simulink model "s20260507_5_PIDAdConfig_IMU_quadleg"  (R2025a)
settings: Solver=FixedStepAuto  StartTime=0.0  StopTime=inf  FixedStep=1/100  RelTol=1e-3
undefined symbols (not defined in the file or in its folder): leg1_config, National_Instruments, PCI
libraries: slpidlib x4, sldrtlib x3, simulink x3, cstblocks x2, hostiolib x1, dspstat3 x1
settings Model: Creator=dperera  LastModifiedBy=dperera
settings RTWCC: GPUComputeCapability=3.5

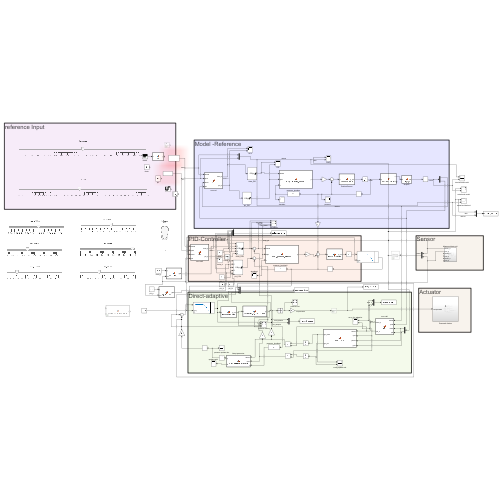
[thumbnail: Simulink's stored preview of the top-level diagram]
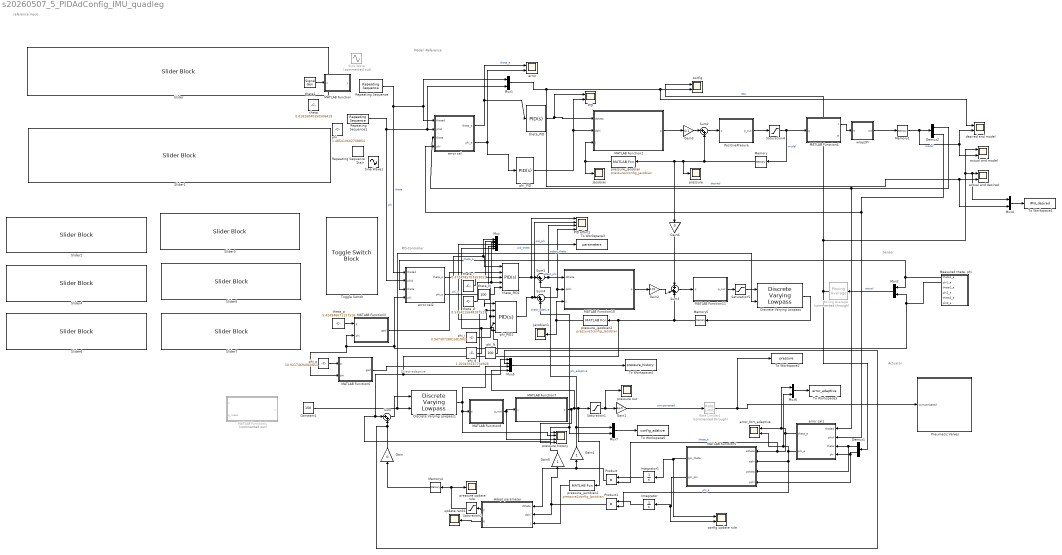
== system s20260507_5_PIDAdConfig_IMU_quadleg ==
  note: reference Input
  note: Actuator
  note: Sensor
  note: Direct-adaptive
  note: PID-Controller
  note: Model -Reference
  Adapt parameter : MATLAB Function  TreatAsAtomicUnit=on
  Constant1 : Constant  Value=150
  Demux1 : Demux  Outputs=2
  Demux2 : Demux  Outputs=2
  Discrete Varying Lowpass : cstblocks/Linear Parameter Varying/Discrete Varying Lowpass  N=1  w0=0  Ts=0.01
  Discrete Varying Lowpass1 : cstblocks/Linear Parameter Varying/Discrete Varying Lowpass  N=1  w0=0  Ts=0.01
  Gain : Gain  Gain=0
  Gain1 : Gain  Gain=1e-5
  Gain2 : Gain  Gain=0.01
  Gain3 : Gain  Gain=0.1
  Gain4 : Gain
  Gain5 : Gain
  Gain6 : Gain  Gain=0
  Integrator : Integrator
  Integrator1 : Integrator
  Jacobian : Scope
      settings: ActiveDisplayYMinimum=-10.825317547305481  ActiveDisplayYMaximum=10.825317547305481  DataLoggingVariableName=ScopeData3
  Jacobian1 : Scope
      settings: ActiveDisplayYMinimum=2.9313515311840069E-6  ActiveDisplayYMaximum=8.8531848611833131E-5  DataLoggingVariableName=ScopeData15
  MATLAB Function : MATLAB Function  TreatAsAtomicUnit=on
  MATLAB Function1 : MATLAB Function  Commented=on  TreatAsAtomicUnit=on
  MATLAB Function10 : MATLAB Function  TreatAsAtomicUnit=on
  MATLAB Function11 : MATLAB Function  TreatAsAtomicUnit=on
  MATLAB Function2 : MATLAB Function  TreatAsAtomicUnit=on
  MATLAB Function3 : MATLAB Function  TreatAsAtomicUnit=on
  MATLAB Function4 : MATLAB Function  TreatAsAtomicUnit=on
  MATLAB Function5 : MATLAB Function  TreatAsAtomicUnit=on
  MATLAB Function6 : MATLAB Function  TreatAsAtomicUnit=on
  MATLAB Function7 : MATLAB Function  TreatAsAtomicUnit=on
  MATLAB Function8 : MATLAB Function  TreatAsAtomicUnit=on
  "Measured theta, phi" : Subsystem
  Memory : Memory  InitialCondition=[1; 1.1; 1]  LinearizeMemory=on  LinearizeAsDelay=on
  Memory1 : Memory  InitialCondition=[0.0001, 0.0001]  LinearizeMemory=on  LinearizeAsDelay=on
  Memory4 : Memory  InitialCondition=[0; 0; 0]
  Memory5 : Memory  InitialCondition=[1; 1.1; 1]  LinearizeMemory=on  LinearizeAsDelay=on
  Moving Average : dspstat3/Moving Average  Commented=through  Method=Sliding window  ForgettingFactorPort=off  SpecifyWindowLength=on  WindowLength=4  OverlapLength=3  AllowArbitraryInputLength=off  ForgettingFactor=0.9  SimulateUsing=Interpreted execution
  Mux : Mux  Inputs=6
  Mux{1..2,4,6..7} (5 alike) : Mux  Inputs=2
  Mux5 : Mux
  PID : Scope  NumInputPorts=2
      settings: ActiveDisplayYMinimum=-3.9804584732791981  ActiveDisplayYMaximum=3.8453740981888478  DataLoggingVariableName=ScopeData4
  PID efforts : Scope  NumInputPorts=4
      settings: ActiveDisplayYMinimum=-41.407944293192642  ActiveDisplayYMaximum=165.36846848361682  DataLoggingVariableName=ScopeData5
  Pneumatic Valves : Subsystem
  PositivePresure : MATLAB Function  TreatAsAtomicUnit=on
  Product : Product
  Product1 : Product
  Rate Limiter1 : RateLimiter  Commented=through  SampleTimeMode=inherited
  Repeating Sequence : simulink/Sources/Repeating Sequence  rep_seq_t=t  rep_seq_y=leg1_config(1,:)
  Repeating Sequence Stair : simulink/Sources/Repeating Sequence Stair  OutValues=[1.1 1.6].'  tsamp=1  OutMin=[]  OutMax=[]  OutDataTypeStr=double  OutputDataTypeScalingMode=double  OutDataType=fixdt(0,8)  ConRadixGroup=Best Precision: Vector-wise  OutScaling=2^-12
  Repeating Sequence1 : simulink/Sources/Repeating Sequence  rep_seq_t=t  rep_seq_y=leg1_config(2,:)
  Saturation{1..2,4..5} (4 alike) : Saturate  UpperLimit=300000  LowerLimit=0
  Sine Wave : Sin  Commented=on  Amplitude=0.2  Frequency=1/2  SampleTime=0
  Sine Wave1 : Sin  Amplitude=1.5/4  Bias=1  Frequency=0.5  SampleTime=0
  Slider : SliderBlock  ScaleMin=-3.14  ScaleMax=3.14
  Slider1 : SliderBlock  ScaleMax=3.14
  Slider2 : SliderBlock  ScaleMax=10
  Slider3 : SliderBlock  ScaleMax=20
  Slider4 : SliderBlock  ScaleMax=1
  Slider5 : SliderBlock  ScaleMax=1
  Slider6 : SliderBlock  ScaleMax=3
  Slider7 : SliderBlock  ScaleMax=3
  Sum{,1..2,4} (4 alike) : Sum  Inputs=|++
  Sum3 : Sum  Inputs=+|++
  To Workspace1 : ToWorkspace  VariableName=IMU_desired  SaveFormat=Timeseries  SampleTime=-1
  To Workspace2 : ToWorkspace  VariableName=pressure  SaveFormat=Timeseries  SampleTime=-1
  To Workspace3 : ToWorkspace  VariableName=parameters  SaveFormat=Timeseries  SampleTime=-1
  To Workspace4 : ToWorkspace  VariableName=pressure_history  SaveFormat=Timeseries  SampleTime=-1
  To Workspace5 : ToWorkspace  VariableName=error_adaptive  SaveFormat=Timeseries  SampleTime=-1
  To Workspace6 : ToWorkspace  VariableName=config_adative  SaveFormat=Timeseries  SampleTime=-1
  Toggle Switch : ToggleSwitchBlock
  actual and desired : Scope  NumInputPorts=2
      settings: ActiveDisplayYMinimum=-3.9267574076576723  ActiveDisplayYMaximum=3.9248901330211212  DataLoggingVariableName=ScopeData8
  actual and model : Scope  NumInputPorts=2
      settings: ActiveDisplayYMinimum=-2.3315152827249515  ActiveDisplayYMaximum=2.6797978799735036  DataLoggingVariableName=ScopeData16
  config : Scope  NumInputPorts=2
      settings: ActiveDisplayYMinimum=-3.926205418823844  ActiveDisplayYMaximum=3.9199222335166648
  config update rule : Scope  NumInputPorts=2
      settings: ActiveDisplayYMinimum=-0.92286339962463748  ActiveDisplayYMaximum=0.53131241193978052  DataLoggingVariableName=ScopeData13
  desired and model : Scope  NumInputPorts=2
      settings: ActiveDisplayYMinimum=-3.9267537424057748  ActiveDisplayYMaximum=3.9248571457540451  DataLoggingVariableName=ScopeData14
  error : Scope  NumInputPorts=2
      settings: ActiveDisplayYMinimum=-1.7062614665873941  ActiveDisplayYMaximum=3.7647403361072445
  error cal : MATLAB Function  TreatAsAtomicUnit=on
  error cal1 : MATLAB Function  TreatAsAtomicUnit=on
  error cal2 : MATLAB Function  TreatAsAtomicUnit=on
  error_fort_adaptive : Scope  NumInputPorts=2
      settings: ActiveDisplayYMinimum=-2.3074635708077071  ActiveDisplayYMaximum=1.3880246681318078  DataLoggingVariableName=ScopeData11
  phi : Constant  Value=1.485410602708854
  phi_N : Constant  Value=100
  phi_PID : slpidlib/PID Controller  Controller=PID  Form=Parallel  TimeDomain=Continuous-time  UseExternalTs=off  SampleTime=-1  IntegratorMethod=Forward Euler  FilterMethod=Forward Euler  ControllerParametersSource=internal  P=10  I=0.5  UseKiTs=off  D=0.01  UseExternalDerivativeSource=off  N=100  UseFilter=on  TunerSelectOption=Transfer Function Based (PID Tuner App)  InitialConditionSource=internal  InitialConditionForIntegrator=0  InitialConditionForFilter=0  DifferentiatorICPrevScaledInput=0  ExternalReset=none  TrackingMode=off  Kt=1  LimitOutput=on  SatLimitsSource=internal  UpperSaturationLimit=inf  LowerSaturationLimit=-inf  LinearizeAsGain=off  AntiWindupMode=back-calculation  Kb=1  LimitIntegrator=off  UpperIntegratorSaturationLimit=10  LowerIntegratorSaturationLimit=-10  POutMin=[]  POutMax=[]  IOutMin=[]  IOutMax=[]  DOutMin=[]  DOutMax=[]  NOutMin=[]  NOutMax=[]  SumOutMin=[]  SumOutMax=[]  SaturationOutMin=[]  SaturationOutMax=[]  PParamMin=[]  PParamMax=[]  IParamMin=[]  IParamMax=[]  DParamMin=[]  DParamMax=[]  NParamMin=[]  NParamMax=[]  KbParamMin=[]  KbParamMax=[]  KtParamMin=[]  KtParamMax=[]  KbOutMin=[]  KbOutMax=[]  KtOutMin=[]  KtOutMax=[]  IntegratorOutMin=[]  IntegratorOutMax=[]  FilterOutMin=[]  FilterOutMax=[]  SumI1OutMin=[]  SumI1OutMax=[]  SumI2OutMin=[]  SumI2OutMax=[]  SumI3OutMin=[]  SumI3OutMax=[]  SumI4OutMin=[]  SumI4OutMax=[]  SumDOutMin=[]  SumDOutMax=[]  DifferentiatorOutMin=[]  DifferentiatorOutMax=[]  FilterDiffOutCoefMin=[]  FilterDiffOutCoefMax=[]  ReciprocalOutMin=[]  ReciprocalOutMax=[]  SumDenOutMin=[]  SumDenOutMax=[]  SumNumOutMin=[]  SumNumOutMax=[]  DivideOutMin=[]  DivideOutMax=[]  UdiffTsProdOutMin=[]  UdiffTsProdOutMax=[]  NTsProdOutMin=[]  NTsProdOutMax=[]  UintegralTsProdOutMin=[]  UintegralTsProdOutMax=[]  UngainTsProdOutMin=[]  UngainTsProdOutMax=[]  ClampingZeroOutDataTypeStr=Inherit: Inherit via back propagation  ClampingZeroOutMin=[]  ClampingZeroOutMax=[]  FilterDenConstantOutDataTypeStr=Inherit: Inherit via back propagation  FilterDenConstantOutMin=[]  FilterDenConstantOutMax=[]  PCopyOutDataTypeStr=Inherit: Inherit via back propagation  PCopyOutMin=[]  PCopyOutMax=[]  NCopyOutDataTypeStr=Inherit: Inherit via back propagation  NCopyOutMin=[]  NCopyOutMax=[]  IntegratorContinuousStateAttributes=''  IntegratorStateMustResolveToSignalObject=off  IntegratorRTWStateStorageClass=Auto  FilterContinuousStateAttributes=''  FilterStateMustResolveToSignalObject=off  FilterRTWStateStorageClass=Auto  ParallelPVariant=InternalParameters  IdealPVariant=Disabled  IVariant=InternalParameters  DVariant=InternalParameters  IntegratorVariant=Continuous  SatVariant=Enabled  AWVariant=BackCalculation  PCopyVariant=Disabled  TRVariant=Disabled  FdbkBlocksVariant=Forward  IdealPFdbkVariant=Disabled  SatFdbkVariant=Disabled  DerivativeFilterVariant=ContFilter  NVariant=InternalParameters  NCopyVariant=Disabled  FilterICVariant=InternalICsFilter  IntegratorICVariant=InternalICs  ExternalResetVariant=Disabled  TRSumVariant=Passthrough  SumFdbkVariant=Disabled  SumVariant=Sum_PID  TsampFilterVariant=InternalTs  TsampNgainVariant=Passthrough  TsampIntegralVariant=Disabled_SignalSpec  ExternalSaturationOutDataTypeStr=Inherit: Same as second input  DerivativeSourceVariant=ErrorSignal  PreIntVariant=InternalPreInt
  phi_PID1 : slpidlib/PID Controller  Controller=PID  Form=Parallel  TimeDomain=Continuous-time  UseExternalTs=off  SampleTime=-1  IntegratorMethod=Forward Euler  FilterMethod=Forward Euler  ControllerParametersSource=external  P=3.5  I=0.01  UseKiTs=off  D=0.02  UseExternalDerivativeSource=off  N=100  UseFilter=on  TunerSelectOption=Transfer Function Based (PID Tuner App)  InitialConditionSource=internal  InitialConditionForIntegrator=0  InitialConditionForFilter=0  DifferentiatorICPrevScaledInput=0  ExternalReset=none  TrackingMode=off  Kt=1  LimitOutput=on  SatLimitsSource=internal  UpperSaturationLimit=inf  LowerSaturationLimit=-inf  LinearizeAsGain=off  AntiWindupMode=back-calculation  Kb=2  LimitIntegrator=off  UpperIntegratorSaturationLimit=10  LowerIntegratorSaturationLimit=-10  POutMin=[]  POutMax=[]  IOutMin=[]  IOutMax=[]  DOutMin=[]  DOutMax=[]  NOutMin=[]  NOutMax=[]  SumOutMin=[]  SumOutMax=[]  SaturationOutMin=[]  SaturationOutMax=[]  PParamMin=[]  PParamMax=[]  IParamMin=[]  IParamMax=[]  DParamMin=[]  DParamMax=[]  NParamMin=[]  NParamMax=[]  KbParamMin=[]  KbParamMax=[]  KtParamMin=[]  KtParamMax=[]  KbOutMin=[]  KbOutMax=[]  KtOutMin=[]  KtOutMax=[]  IntegratorOutMin=[]  IntegratorOutMax=[]  FilterOutMin=[]  FilterOutMax=[]  SumI1OutMin=[]  SumI1OutMax=[]  SumI2OutMin=[]  SumI2OutMax=[]  SumI3OutMin=[]  SumI3OutMax=[]  SumI4OutMin=[]  SumI4OutMax=[]  SumDOutMin=[]  SumDOutMax=[]  DifferentiatorOutMin=[]  DifferentiatorOutMax=[]  FilterDiffOutCoefMin=[]  FilterDiffOutCoefMax=[]  ReciprocalOutMin=[]  ReciprocalOutMax=[]  SumDenOutMin=[]  SumDenOutMax=[]  SumNumOutMin=[]  SumNumOutMax=[]  DivideOutMin=[]  DivideOutMax=[]  UdiffTsProdOutMin=[]  UdiffTsProdOutMax=[]  NTsProdOutMin=[]  NTsProdOutMax=[]  UintegralTsProdOutMin=[]  UintegralTsProdOutMax=[]  UngainTsProdOutMin=[]  UngainTsProdOutMax=[]  ClampingZeroOutDataTypeStr=Inherit: Inherit via back propagation  ClampingZeroOutMin=[]  ClampingZeroOutMax=[]  FilterDenConstantOutDataTypeStr=Inherit: Inherit via back propagation  FilterDenConstantOutMin=[]  FilterDenConstantOutMax=[]  PCopyOutDataTypeStr=Inherit: Inherit via back propagation  PCopyOutMin=[]  PCopyOutMax=[]  NCopyOutDataTypeStr=Inherit: Inherit via back propagation  NCopyOutMin=[]  NCopyOutMax=[]  IntegratorContinuousStateAttributes=''  IntegratorStateMustResolveToSignalObject=off  IntegratorRTWStateStorageClass=Auto  FilterContinuousStateAttributes=''  FilterStateMustResolveToSignalObject=off  FilterRTWStateStorageClass=Auto  ParallelPVariant=ExternalParameters  IdealPVariant=Disabled  IVariant=ExternalParameters  DVariant=ExternalParameters  IntegratorVariant=Continuous  SatVariant=Enabled  AWVariant=BackCalculation  PCopyVariant=Disabled  TRVariant=Disabled  FdbkBlocksVariant=Forward  IdealPFdbkVariant=Disabled  SatFdbkVariant=Disabled  DerivativeFilterVariant=ContFilter  NVariant=ExternalParameters  NCopyVariant=Disabled  FilterICVariant=InternalICsFilter  IntegratorICVariant=InternalICs  ExternalResetVariant=Disabled  TRSumVariant=Passthrough  SumFdbkVariant=Disabled  SumVariant=Sum_PID  TsampFilterVariant=InternalTs  TsampNgainVariant=Passthrough  TsampIntegralVariant=Disabled_SignalSpec  ExternalSaturationOutDataTypeStr=Inherit: Same as second input  DerivativeSourceVariant=ErrorSignal  PreIntVariant=InternalPreInt
  phi_d : Constant  Value=1.020433147734928
  phi_i : Constant  Value=0.9473072881581902
  phi_p : Constant  Value=10.92174694060851
  pressure : Scope
      settings: ActiveDisplayYMinimum=-37499.999999999993  ActiveDisplayYMaximum=337500  DataLoggingVariableName=ScopeData2
  pressure history : Scope  NumInputPorts=4
      settings: ActiveDisplayYMinimum=-38849.124995166283  ActiveDisplayYMaximum=349642.12495649664  DataLoggingVariableName=ScopeData17
  pressure out : Scope
      settings: ActiveDisplayYMinimum=-37499.999999999993  ActiveDisplayYMaximum=337500  DataLoggingVariableName=ScopeData12
  pressure update rule : Scope
      settings: ActiveDisplayYMinimum=-11428.615964886589  ActiveDisplayYMaximum=102857.54368397931  DataLoggingVariableName=ScopeData9
  pressure_jacobian : MATLABFcn  MATLABFcn=pressure2config_Jacobian  OutputDimensions=[2 3]  OutputSignalType=real  Output1D=off
  pressure_jacobian1 : MATLABFcn  MATLABFcn=pressure2config_Jacobian  OutputDimensions=[2 3]  OutputSignalType=real  Output1D=off
  pressure_jacobian2 : MATLABFcn  MATLABFcn=pressure2config_Jacobian  OutputDimensions=[2 3]  OutputSignalType=real  Output1D=off
  theta : Constant  Value=0.01826040350506419
  theta1 : SignalGenerator  WaveForm=sawtooth  Amplitude=pi  Frequency=0.05*2*pi  Units=rad/sec  VectorParams1D=off
  theta_N : Constant  Value=100
  theta_PID : slpidlib/PID Controller  Controller=PID  Form=Parallel  TimeDomain=Continuous-time  UseExternalTs=off  SampleTime=-1  IntegratorMethod=Forward Euler  FilterMethod=Forward Euler  ControllerParametersSource=internal  P=5  I=0.1  UseKiTs=off  D=0  UseExternalDerivativeSource=off  N=100  UseFilter=on  TunerSelectOption=Transfer Function Based (PID Tuner App)  InitialConditionSource=internal  InitialConditionForIntegrator=0  InitialConditionForFilter=0  DifferentiatorICPrevScaledInput=0  ExternalReset=none  TrackingMode=off  Kt=1  LimitOutput=on  SatLimitsSource=internal  UpperSaturationLimit=inf  LowerSaturationLimit=-inf  LinearizeAsGain=off  AntiWindupMode=back-calculation  Kb=1  LimitIntegrator=off  UpperIntegratorSaturationLimit=10  LowerIntegratorSaturationLimit=-10  POutMin=[]  POutMax=[]  IOutMin=[]  IOutMax=[]  DOutMin=[]  DOutMax=[]  NOutMin=[]  NOutMax=[]  SumOutMin=[]  SumOutMax=[]  SaturationOutMin=[]  SaturationOutMax=[]  PParamMin=[]  PParamMax=[]  IParamMin=[]  IParamMax=[]  DParamMin=[]  DParamMax=[]  NParamMin=[]  NParamMax=[]  KbParamMin=[]  KbParamMax=[]  KtParamMin=[]  KtParamMax=[]  KbOutMin=[]  KbOutMax=[]  KtOutMin=[]  KtOutMax=[]  IntegratorOutMin=[]  IntegratorOutMax=[]  FilterOutMin=[]  FilterOutMax=[]  SumI1OutMin=[]  SumI1OutMax=[]  SumI2OutMin=[]  SumI2OutMax=[]  SumI3OutMin=[]  SumI3OutMax=[]  SumI4OutMin=[]  SumI4OutMax=[]  SumDOutMin=[]  SumDOutMax=[]  DifferentiatorOutMin=[]  DifferentiatorOutMax=[]  FilterDiffOutCoefMin=[]  FilterDiffOutCoefMax=[]  ReciprocalOutMin=[]  ReciprocalOutMax=[]  SumDenOutMin=[]  SumDenOutMax=[]  SumNumOutMin=[]  SumNumOutMax=[]  DivideOutMin=[]  DivideOutMax=[]  UdiffTsProdOutMin=[]  UdiffTsProdOutMax=[]  NTsProdOutMin=[]  NTsProdOutMax=[]  UintegralTsProdOutMin=[]  UintegralTsProdOutMax=[]  UngainTsProdOutMin=[]  UngainTsProdOutMax=[]  ClampingZeroOutDataTypeStr=Inherit: Inherit via back propagation  ClampingZeroOutMin=[]  ClampingZeroOutMax=[]  FilterDenConstantOutDataTypeStr=Inherit: Inherit via back propagation  FilterDenConstantOutMin=[]  FilterDenConstantOutMax=[]  PCopyOutDataTypeStr=Inherit: Inherit via back propagation  PCopyOutMin=[]  PCopyOutMax=[]  NCopyOutDataTypeStr=Inherit: Inherit via back propagation  NCopyOutMin=[]  NCopyOutMax=[]  IntegratorContinuousStateAttributes=''  IntegratorStateMustResolveToSignalObject=off  IntegratorRTWStateStorageClass=Auto  FilterContinuousStateAttributes=''  FilterStateMustResolveToSignalObject=off  FilterRTWStateStorageClass=Auto  ParallelPVariant=InternalParameters  IdealPVariant=Disabled  IVariant=InternalParameters  DVariant=InternalParameters  IntegratorVariant=Continuous  SatVariant=Enabled  AWVariant=BackCalculation  PCopyVariant=Disabled  TRVariant=Disabled  FdbkBlocksVariant=Forward  IdealPFdbkVariant=Disabled  SatFdbkVariant=Disabled  DerivativeFilterVariant=ContFilter  NVariant=InternalParameters  NCopyVariant=Disabled  FilterICVariant=InternalICsFilter  IntegratorICVariant=InternalICs  ExternalResetVariant=Disabled  TRSumVariant=Passthrough  SumFdbkVariant=Disabled  SumVariant=Sum_PID  TsampFilterVariant=InternalTs  TsampNgainVariant=Passthrough  TsampIntegralVariant=Disabled_SignalSpec  ExternalSaturationOutDataTypeStr=Inherit: Same as second input  DerivativeSourceVariant=ErrorSignal  PreIntVariant=InternalPreInt
  theta_PID1 : slpidlib/PID Controller  Controller=PID  Form=Parallel  TimeDomain=Continuous-time  UseExternalTs=off  SampleTime=-1  IntegratorMethod=Forward Euler  FilterMethod=Forward Euler  ControllerParametersSource=external  P=3  I=0.1  UseKiTs=off  D=0.001  UseExternalDerivativeSource=off  N=100  UseFilter=on  TunerSelectOption=Transfer Function Based (PID Tuner App)  InitialConditionSource=internal  InitialConditionForIntegrator=0  InitialConditionForFilter=0  DifferentiatorICPrevScaledInput=0  ExternalReset=none  TrackingMode=off  Kt=1  LimitOutput=on  SatLimitsSource=internal  UpperSaturationLimit=inf  LowerSaturationLimit=-inf  LinearizeAsGain=off  AntiWindupMode=back-calculation  Kb=2  LimitIntegrator=off  UpperIntegratorSaturationLimit=10  LowerIntegratorSaturationLimit=-10  POutMin=[]  POutMax=[]  IOutMin=[]  IOutMax=[]  DOutMin=[]  DOutMax=[]  NOutMin=[]  NOutMax=[]  SumOutMin=[]  SumOutMax=[]  SaturationOutMin=[]  SaturationOutMax=[]  PParamMin=[]  PParamMax=[]  IParamMin=[]  IParamMax=[]  DParamMin=[]  DParamMax=[]  NParamMin=[]  NParamMax=[]  KbParamMin=[]  KbParamMax=[]  KtParamMin=[]  KtParamMax=[]  KbOutMin=[]  KbOutMax=[]  KtOutMin=[]  KtOutMax=[]  IntegratorOutMin=[]  IntegratorOutMax=[]  FilterOutMin=[]  FilterOutMax=[]  SumI1OutMin=[]  SumI1OutMax=[]  SumI2OutMin=[]  SumI2OutMax=[]  SumI3OutMin=[]  SumI3OutMax=[]  SumI4OutMin=[]  SumI4OutMax=[]  SumDOutMin=[]  SumDOutMax=[]  DifferentiatorOutMin=[]  DifferentiatorOutMax=[]  FilterDiffOutCoefMin=[]  FilterDiffOutCoefMax=[]  ReciprocalOutMin=[]  ReciprocalOutMax=[]  SumDenOutMin=[]  SumDenOutMax=[]  SumNumOutMin=[]  SumNumOutMax=[]  DivideOutMin=[]  DivideOutMax=[]  UdiffTsProdOutMin=[]  UdiffTsProdOutMax=[]  NTsProdOutMin=[]  NTsProdOutMax=[]  UintegralTsProdOutMin=[]  UintegralTsProdOutMax=[]  UngainTsProdOutMin=[]  UngainTsProdOutMax=[]  ClampingZeroOutDataTypeStr=Inherit: Inherit via back propagation  ClampingZeroOutMin=[]  ClampingZeroOutMax=[]  FilterDenConstantOutDataTypeStr=Inherit: Inherit via back propagation  FilterDenConstantOutMin=[]  FilterDenConstantOutMax=[]  PCopyOutDataTypeStr=Inherit: Inherit via back propagation  PCopyOutMin=[]  PCopyOutMax=[]  NCopyOutDataTypeStr=Inherit: Inherit via back propagation  NCopyOutMin=[]  NCopyOutMax=[]  IntegratorContinuousStateAttributes=''  IntegratorStateMustResolveToSignalObject=off  IntegratorRTWStateStorageClass=Auto  FilterContinuousStateAttributes=''  FilterStateMustResolveToSignalObject=off  FilterRTWStateStorageClass=Auto  ParallelPVariant=ExternalParameters  IdealPVariant=Disabled  IVariant=ExternalParameters  DVariant=ExternalParameters  IntegratorVariant=Continuous  SatVariant=Enabled  AWVariant=BackCalculation  PCopyVariant=Disabled  TRVariant=Disabled  FdbkBlocksVariant=Forward  IdealPFdbkVariant=Disabled  SatFdbkVariant=Disabled  DerivativeFilterVariant=ContFilter  NVariant=ExternalParameters  NCopyVariant=Disabled  FilterICVariant=InternalICsFilter  IntegratorICVariant=InternalICs  ExternalResetVariant=Disabled  TRSumVariant=Passthrough  SumFdbkVariant=Disabled  SumVariant=Sum_PID  TsampFilterVariant=InternalTs  TsampNgainVariant=Passthrough  TsampIntegralVariant=Disabled_SignalSpec  ExternalSaturationOutDataTypeStr=Inherit: Same as second input  DerivativeSourceVariant=ErrorSignal  PreIntVariant=InternalPreInt
  theta_d : Constant  Value=0.5354215648287513
  theta_i : Constant  Value=0.3724785703353051
  theta_p : Constant  Value=5.424946671157516
  update rank1 : Scope
      settings: ActiveDisplayYMinimum=-0.12499999999999997  ActiveDisplayYMaximum=1.125  DataLoggingVariableName=ScopeData10
  wrap2Pi : MATLAB Function  TreatAsAtomicUnit=on
  wires:
  error cal/2(phi_e) -> error/2, phi_PID/1
  pressure_jacobian/1 -> Jacobian/1, MATLAB Function2/3(J)
  theta_PID/1 -> PID/1, MATLAB Function2/1(dtheta)
  phi_PID/1 -> PID/2, MATLAB Function2/2(dphi)
  Memory/1 -> pressure/1, Gain6/1, pressure_jacobian/1, Sum2/2
  Mux1/1 -> desired and model/1, config/2, Mux4/2, actual and desired/2  "desired"
  Gain3/1 -> Sum2/1
  Sum2/1 -> PositivePresure/1(p)
  Saturation4/1 -> MATLAB Function4/1(p), Memory/1  "model"
  MATLAB Function2/1(p) -> Gain3/1
  error cal/1(theta_e) -> error/1, theta_PID/1  "theta_e"
  Mux2/1 -> Moving Average/1  "actual"
  theta1/1 -> MATLAB Function/1(u)
  PositivePresure/1(p_out) -> Saturation4/1
  Integrator1/1 -> Product/1
  Integrator/1 -> Product1/1
  Adapt parameter/1(p) -> Saturation2/1
  Saturation2/1 -> Memory4/1, pressure update rule/1
  error cal1/2(phi_e) -> error_fort_adaptive/2, Mux6/2, Product1/2, MATLAB Function5/2(ephi)  "phi_e"
  pressure_jacobian1/1 -> Adapt parameter/3(J)
  MATLAB Function5/2(gm_phi) -> config update rule/2, Integrator/1
  Product/1 -> Adapt parameter/1(dtheta), Gain4/1
  Demux2/2 -> error cal1/2(phid), error cal/4(phi)
  error cal1/1(theta_e) -> Mux6/1, error_fort_adaptive/1, Product/2, MATLAB Function5/1(etheta)  "theta_e"
  Demux2/1 -> error cal1/1(thetad), error cal/3(theta)
  Product1/1 -> Gain5/1, Adapt parameter/2(dphi)
  Demux1/2 -> MATLAB Function5/4(pphi), error cal1/4(phi)
  Sum/1 -> Discrete Varying Lowpass1/1
  Demux1/1 -> MATLAB Function5/3(ptheta), error cal1/3(theta)
  Gain/1 -> Mux5/2, Sum/2
  Adapt parameter/2(R) -> update rank1/1
  MATLAB Function5/1(gm_theta) -> Integrator1/1, config update rule/1
  wrap2Pi/1(wa) -> Memory1/1
  MATLAB Function4/1(c) -> wrap2Pi/1(a)
  Saturation1/1 -> pressure out/1, Gain1/1
  Gain1/1 -> Rate Limiter1/1  "compensated"
  Memory1/1 -> actual and model/2, desired and model/2, Demux2/1  "model"
  Memory4/1 -> Gain/1
  MATLAB Function11/1(p_out) -> Saturation5/1
  "Measured theta, phi"/1(theta1_a) -> Mux2/1, error cal2/3(theta)
  MATLAB Function10/1(p) -> Gain2/1
  phi_PID1/1 -> PID efforts/2, Sum4/1  "pid_phi"
  error cal2/2(phi_e) -> phi_PID1/1  "phi_e"
  "Measured theta, phi"/2(phi1_a) -> Mux2/2, MATLAB Function6/2(phi), MATLAB Function3/2(phi), error cal2/4(phi)
  Memory5/1 -> Sum3/3, pressure_jacobian2/1, pressure history/1, Sum/1, Mux5/1
  Sum3/1 -> MATLAB Function11/1(p)
  Repeating Sequence/1 -> error cal2/1(thetad), error cal/1(thetad), Mux1/1  "theta"
  pressure_jacobian2/1 -> Jacobian1/1, MATLAB Function10/3(J)
  Saturation5/1 -> Discrete Varying Lowpass/1
  Repeating Sequence1/1 -> error cal2/2(phid), Mux1/2, error cal/2(phid)  "phi"
  error cal2/1(theta_e) -> Mux/1, theta_PID1/1  "theta_e"
  MATLAB Function7/1(p) -> Mux5/4, pressure_jacobian1/1, Saturation1/1, pressure history/4
  MATLAB Function8/1(p_out) -> MATLAB Function7/1(x), pressure history/3
  Moving Average/1 -> actual and model/1, Mux4/1, actual and desired/1, config/1, Demux1/1  "IMU"
  Mux4/1 -> To Workspace1/1
  MATLAB Function6/1(gad) -> Mux/4, phi_PID1/2
  phi_i/1 -> Mux/5, phi_PID1/3
  phi_d/1 -> phi_PID1/4, Mux/6
  phi_N/1 -> phi_PID1/5
  MATLAB Function3/1(gad) -> theta_PID1/2
  theta_i/1 -> Mux/2, theta_PID1/3
  theta_d/1 -> Mux/3, theta_PID1/4
  theta_N/1 -> theta_PID1/5
  theta_p/1 -> MATLAB Function3/1(g)
  phi_p/1 -> MATLAB Function6/1(g)
  Discrete Varying Lowpass/1 -> Memory5/1
  Rate Limiter1/1 -> To Workspace2/1, Pneumatic Valves/1(compensated)
  Mux/1 -> To Workspace3/1
  Mux5/1 -> To Workspace4/1
  theta_PID1/1 -> PID efforts/1, Sum1/1  "pid_theta"
  Sum1/1 -> PID efforts/3, MATLAB Function10/1(dtheta)  "adapt_theta"
  Sum4/1 -> PID efforts/4, MATLAB Function10/2(dphi)  "adapt_phi"
  Gain4/1 -> Mux7/1, Sum1/2  "theta_adative"
  Gain5/1 -> Mux7/2, Sum4/2  "phi_adaptive"
  Constant1/1 -> Discrete Varying Lowpass/2, Discrete Varying Lowpass1/2
  Discrete Varying Lowpass1/1 -> Mux5/3, pressure history/2, MATLAB Function8/1(p)
  Gain2/1 -> Sum3/2
  Gain6/1 -> Sum3/1
  Mux6/1 -> To Workspace5/1
  Mux7/1 -> To Workspace6/1

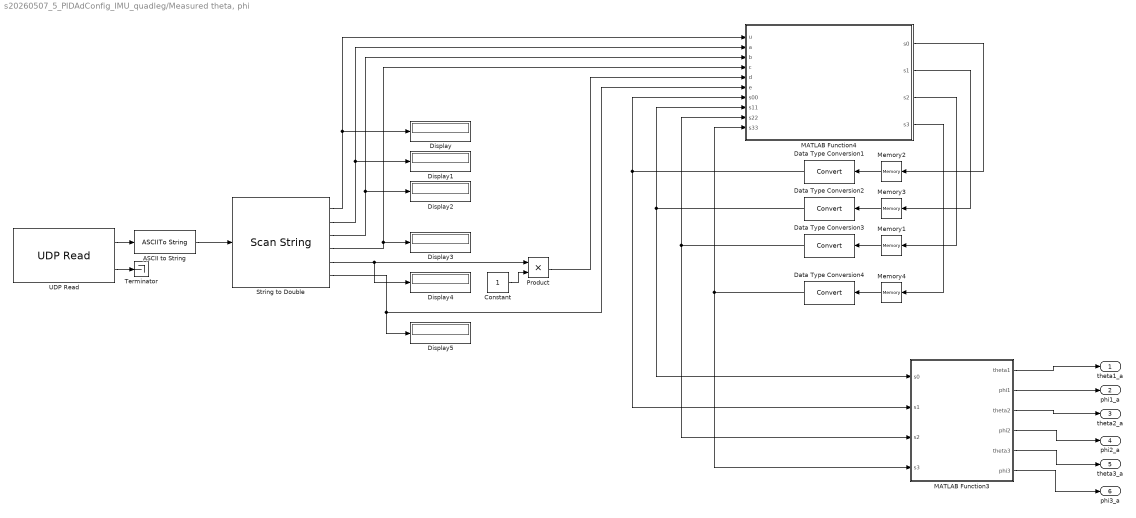
== system s20260507_5_PIDAdConfig_IMU_quadleg/Measured theta, phi ==
  ASCII to String : ASCIIToString
  Constant : Constant
  Data Type Conversion{1..4} (4 alike) : DataTypeConversion  SaturateOnIntegerOverflow=off  RndMeth=Floor
  Display{,1..5} (6 alike) : Display
  MATLAB Function3 : MATLAB Function  TreatAsAtomicUnit=on
  MATLAB Function4 : MATLAB Function  TreatAsAtomicUnit=on
  Memory1 : Memory  InitialCondition=[1.0,0,0,0,0,1]  InheritSampleTime=on
  Memory2 : Memory  InitialCondition=[0.0,0,0,0,0,1]  InheritSampleTime=on
  Memory3 : Memory  InitialCondition=[1.0,0,0,0,0,1]  InheritSampleTime=on
  Memory4 : Memory  InitialCondition=[1.0,0,0,0,0,1]  InheritSampleTime=on
  Product : Product
  String to Double : ScanString  Format="\"%f %f %f %f %f %f\""
  Terminator : Terminator
  UDP Read : hostiolib/UDP Read  localURL='0.0.0.0'  localPort=60002  remoteURL='localhost'  remotePort=-1  recvBufferSize=1024  dims=255  signalDatatype=uint8  isVarSize=off  showBlockingTime=on  blockingTime=0  sampletime=0.01  blockPlatform=HOST  hoistedMaskSrc=UDP Read/UDP Read Sim/UDP Read
  theta1_a : Outport
  phi1_a : Outport  Port=2
  theta2_a : Outport  Port=3
  phi2_a : Outport  Port=4
  theta3_a : Outport  Port=5
  phi3_a : Outport  Port=6
  wires:
  ASCII to String/1 -> String to Double/1
  Memory4/1 -> Data Type Conversion4/1
  Constant/1 -> Product/2
  UDP Read/2 -> Terminator/1
  UDP Read/1 -> ASCII to String/1
  String to Double/2 -> MATLAB Function4/2(a), Display1/1
  String to Double/1 -> Display/1, MATLAB Function4/1(u)
  MATLAB Function4/3(s2) -> Memory1/1
  Data Type Conversion4/1 -> MATLAB Function3/4(s3), MATLAB Function4/10(s33)
  String to Double/6 -> Display5/1, MATLAB Function4/6(e)
  Product/1 -> MATLAB Function4/5(d)
  String to Double/4 -> MATLAB Function4/4(c), Display3/1
  String to Double/5 -> Display4/1, Product/1
  Memory2/1 -> Data Type Conversion1/1
  Data Type Conversion2/1 -> MATLAB Function3/1(s0), MATLAB Function4/8(s11)
  Memory1/1 -> Data Type Conversion3/1
  MATLAB Function4/4(s3) -> Memory4/1
  MATLAB Function4/2(s1) -> Memory3/1
  Data Type Conversion3/1 -> MATLAB Function3/3(s2), MATLAB Function4/9(s22)
  Memory3/1 -> Data Type Conversion2/1
  MATLAB Function4/1(s0) -> Memory2/1
  Data Type Conversion1/1 -> MATLAB Function3/2(s1), MATLAB Function4/7(s00)
  String to Double/3 -> MATLAB Function4/3(b), Display2/1
  MATLAB Function3/1(theta1) -> theta1_a/1
  MATLAB Function3/2(phi1) -> phi1_a/1
  MATLAB Function3/3(theta2) -> theta2_a/1
  MATLAB Function3/4(phi2) -> phi2_a/1
  MATLAB Function3/5(theta3) -> theta3_a/1
  MATLAB Function3/6(phi3) -> phi3_a/1

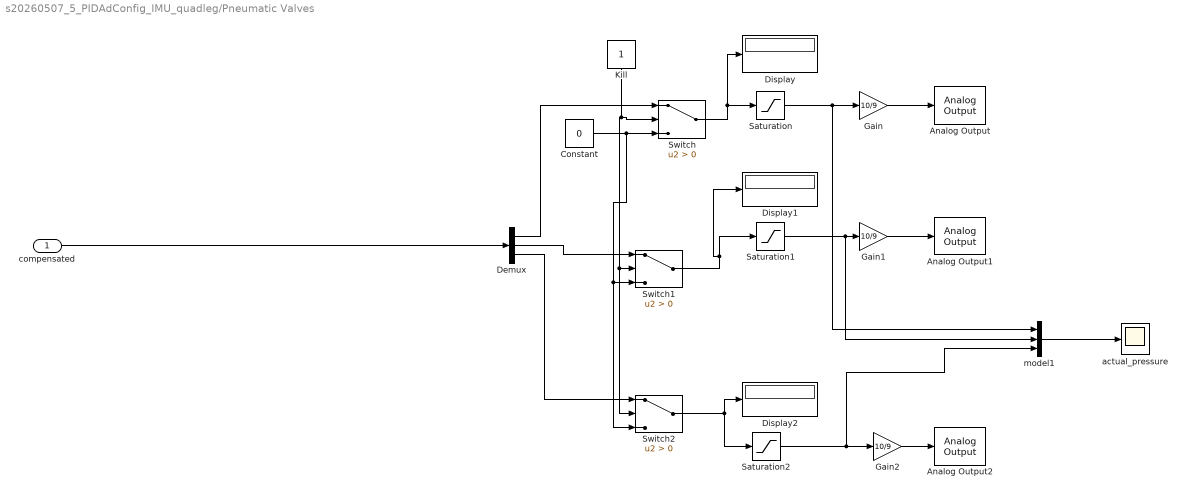
== system s20260507_5_PIDAdConfig_IMU_quadleg/Pneumatic Valves ==
  compensated : Inport
  Analog Output : sldrtlib/Analog Output  SampleTime=1/100  MaxMissedTicks=inf  ShowMissedTicks=off  YieldWhenWaiting=off  DrvName=National_Instruments/PCI-6703  DrvAddress=4294967295  DrvOptions=0  Channels=1  RangeMode=1  VoltRange=1  InitialValue=0  FinalValue=0
      settings: AttributesFormatString=National Instruments\nPCI-6703 [auto]
  Analog Output1 : sldrtlib/Analog Output  SampleTime=1/100  MaxMissedTicks=inf  ShowMissedTicks=off  YieldWhenWaiting=off  DrvName=National_Instruments/PCI-6703  DrvAddress=4294967295  DrvOptions=0  Channels=2  RangeMode=1  VoltRange=1  InitialValue=0  FinalValue=0
      settings: AttributesFormatString=National Instruments\nPCI-6703 [auto]
  Analog Output2 : sldrtlib/Analog Output  SampleTime=1/100  MaxMissedTicks=inf  ShowMissedTicks=off  YieldWhenWaiting=off  DrvName=National_Instruments/PCI-6703  DrvAddress=4294967295  DrvOptions=0  Channels=3  RangeMode=1  VoltRange=1  InitialValue=0  FinalValue=0
      settings: AttributesFormatString=National Instruments\nPCI-6703 [auto]
  Constant : Constant  Value=0
  Demux : Demux  Outputs=3
  Display : Display
  Display1 : Display
  Display2 : Display
  Gain : Gain  Gain=10/9
  Gain1 : Gain  Gain=10/9
  Gain2 : Gain  Gain=10/9
  Kill : Constant
  Saturation : Saturate  UpperLimit=3  LowerLimit=0
  Saturation1 : Saturate  UpperLimit=3  LowerLimit=0
  Saturation2 : Saturate  UpperLimit=3  LowerLimit=0
  Switch : Switch  Criteria=u2 > Threshold  SaturateOnIntegerOverflow=off  InputSameDT=off
  Switch1 : Switch  Criteria=u2 > Threshold  SaturateOnIntegerOverflow=off  InputSameDT=off
  Switch2 : Switch  Criteria=u2 > Threshold  SaturateOnIntegerOverflow=off  InputSameDT=off
  actual_pressure : Scope
      settings: ActiveDisplayYMinimum=-0.37499999999999989  ActiveDisplayYMaximum=3.375  DataLoggingVariableName=ScopeData7
  model1 : Mux  Inputs=3
  wires:
  Constant/1 -> Switch2/3, Switch1/3, Switch/3
  Kill/1 -> Switch2/2, Switch1/2, Switch/2
  Switch/1 -> Display/1, Saturation/1
  Gain/1 -> Analog Output/1
  Saturation/1 -> model1/1, Gain/1
  Demux/3 -> Switch2/1
  Gain1/1 -> Analog Output1/1
  Gain2/1 -> Analog Output2/1
  Saturation2/1 -> model1/3, Gain2/1
  Switch2/1 -> Saturation2/1, Display2/1
  Demux/2 -> Switch1/1
  Switch1/1 -> Saturation1/1, Display1/1
  model1/1 -> actual_pressure/1
  Saturation1/1 -> model1/2, Gain1/1
  Demux/1 -> Switch/1
  compensated/1 -> Demux/1

== matlab function s20260507_5_PIDAdConfig_IMU_quadleg/MATLAB Function5 ==
  data: etheta input; gm_theta output; ephi input; ptheta input; pphi input; gm_phi output
function [gm_theta, gm_phi] = directAdapt(etheta, ephi, ptheta, pphi)
%#codegen

MAX_GM = 100;
DEAD_E = 1e-6;

if ~isfinite(etheta) || ~isfinite(ephi) || ~isfinite(ptheta) || ~isfinite(pphi)
    gm_theta = 0;
    gm_phi   = 0;
    return;
end

if abs(etheta) < DEAD_E
    etheta = 0;
end
if abs(ephi) < DEAD_E
    ephi = 0;
end

gm_theta = -(etheta * ptheta) / (1 + ptheta^2);
gm_phi   = -(ephi   * pphi)   / (1 + pphi^2);

if ~isfinite(gm_theta)
    gm_theta = 0;
else
    gm_theta = min(max(gm_theta, -MAX_GM), MAX_GM);
end

if ~isfinite(gm_phi)
    gm_phi = 0;
else
    gm_phi = min(max(gm_phi, -MAX_GM), MAX_GM);
end

end

== matlab function s20260507_5_PIDAdConfig_IMU_quadleg/MATLAB Function ==
  data: u input; y output
function y = fcn(u)

y = wrapToPi(u - pi);

== matlab function s20260507_5_PIDAdConfig_IMU_quadleg/MATLAB Function11 ==
  data: p input; p_out output
function p_out  = PositivePressure(p)

    minP = min(p);
    maxP = max(p);
    
    p_pos = p-minP;
    % p_pos_norm = p_pos / (maxP - minP) * maxP; % Normalize the positive pressures
    
    p_out = p_pos/max(p_pos) * maxP;
    
end

== matlab function s20260507_5_PIDAdConfig_IMU_quadleg/error cal2 ==
  data: thetad input; theta_e output; phid input; theta input; phi input; phi_e output
function [theta_e, phi_e]    = fcn(thetad, phid, theta, phi)

    % qd = [thetad;phid];
    % q = [theta;phi];
    % 
    % abs_diff = abs(thetad-theta);
    % abs_diff_mod = abs(mod(thetad, 2*pi)-mod(theta, 2*pi));
    % 
    % if abs_diff < abs_diff_mod
    %     error = qd-q;
    % else
    %     error = mod(qd, 2*pi) - mod(q,2*pi);
    % end
    % 
    % if error(1) < 0.0001
    %     error(1) = 0;
    % end
    % 
    % if error(2) < 0.0001
    %     error(2) = 0;
    % end
    % 
    % theta_e = error(1);
    % phi_e = error(2);

        % Compute signed angular differences in (-pi, pi]
    theta_e = atan2(sin(thetad - theta), cos(thetad - theta));
    phi_e   = atan2(sin(phid - phi), cos(phid - phi));

    % Optional: zero small errors
    if abs(theta_e) < 1e-4
        theta_e = 0;
    end
    if abs(phi_e) < 1e-4
        phi_e = 0;
    end

end

== matlab function s20260507_5_PIDAdConfig_IMU_quadleg/error cal1 ==
  data: thetad input; theta_e output; phid input; theta input; phi input; phi_e output
function [theta_e, phi_e]    = fcn(thetad, phid, theta, phi)

    % qd = [thetad;phid];
    % q = [theta;phi];
    % 
    % abs_diff = abs(thetad-theta);
    % abs_diff_mod = abs(mod(thetad, 2*pi)-mod(theta, 2*pi));
    % 
    % if abs_diff < abs_diff_mod
    %     error = qd-q;
    % else
    %     error = mod(qd, 2*pi) - mod(q,2*pi);
    % end
    % 
    % if error(1) < 0.0001
    %     error(1) = 0;
    % end
    % 
    % if error(2) < 0.0001
    %     error(2) = 0;
    % end
    % 
    % theta_e = error(1);
    % phi_e = error(2);

        % Compute signed angular differences in (-pi, pi]
    theta_e = atan2(sin(theta - thetad), cos(theta - thetad));
    phi_e   = atan2(sin(phi - phid), cos(phi - phid));

    % Optional: zero small errors
    if abs(theta_e) < 1e-4
        theta_e = 0;
    end
    if abs(phi_e) < 1e-4
        phi_e = 0;
    end

end

== matlab function s20260507_5_PIDAdConfig_IMU_quadleg/MATLAB Function1 ==
  data: x input; u output; p_meas input
function u = invDeadzone_asymmetric(x, p_meas)
%#codegen
% x      : 3x1 desired effective pressure command
% p_meas : 3x1 measured chamber pressure (preferred)
% u      : 3x1 compensated command to valve/actuator

persistent x_prev u_prev mode ready_count
if isempty(x_prev)
    x_prev      = zeros(3,1);
    u_prev      = zeros(3,1);
    mode        = zeros(3,1);   % 0: hold, 1: load, 2: unload, 3: ready
    ready_count = zeros(3,1);
end

% ---- parameters ----
Pmax    = 3e5 * ones(3,1);
D       = 0.5e5 * ones(3,1);     % deadzone threshold
Dready  = 0.45e5 * ones(3,1);    % keep below D, not exactly at D
d       = 0.1e5 * ones(3,1);     % small transition width

Ts      = 0.01;                 % sample time
du_max  = 6e5;                   % max command slew rate [units/s]

x_eps   = 200;                   % near-zero desired command threshold
dx_eps  = 100;                   % direction detection threshold
p_eps   = 1000;                  % near-zero measured pressure threshold
Nready  = 20;                    % dwell samples before entering READY

u = zeros(3,1);

for i = 1:3
    xi  = x(i);
    pi  = p_meas(i);
    dxi = xi - x_prev(i);

    % ---- mode logic ----
    if dxi > dx_eps
        mode(i) = 1;  % LOAD
        ready_count(i) = 0;
    elseif dxi < -dx_eps
        mode(i) = 2;  % UNLOAD
        ready_count(i) = 0;
    elseif abs(xi) <= x_eps && abs(pi) <= p_eps
        ready_count(i) = ready_count(i) + 1;
        if ready_count(i) >= Nready
            mode(i) = 3;  % READY
        end
    else
        ready_count(i) = 0;
    end

    % ---- desired compensated output ----
    switch mode(i)
        case 1  % LOAD
            u_des = loadingMap(xi, D(i), Dready(i), d(i), Pmax(i));

        case 2  % UNLOAD
            u_des = unloadingMap(xi, Pmax(i));

        case 3  % READY
            u_des = Dready(i);

        otherwise
            u_des = u_prev(i);
    end

    % ---- rate limit ----
    du = u_des - u_prev(i);
    du = min(max(du, -du_max*Ts), du_max*Ts);

    u(i) = u_prev(i) + du;

    % ---- clamp ----
    if u(i) < 0
        u(i) = 0;
    elseif u(i) > Pmax(i)
        u(i) = Pmax(i);
    end
end

x_prev = x;
u_prev = u;


function y = loadingMap(x, D, Dready, d, Pmax)
% Smooth loading map:
% below d, move smoothly from Dready toward D
% above d, continue with affine map

if x <= 0
    y = 0;
elseif x < d
    s = x / d;
    s = s*s*(3 - 2*s);   % smoothstep
    y = Dready + (D - Dready)*s;
else
    y = D + (Pmax - D) * (x - d) / max(Pmax - d, 1e-9);
    if y > Pmax
        y = Pmax;
    end
end


function y = unloadingMap(x, Pmax)
% Simple unloading model.
% Replace this with your identified unloading fit if needed.

if x <= 0
    y = 0;
elseif x >= Pmax
    y = Pmax;
else
    y = x;   % approximately linear unloading
end

== matlab function s20260507_5_PIDAdConfig_IMU_quadleg/MATLAB Function8 ==
  data: p input; p_out output
function p_out  = PositivePressure(p)

    minP = min(p);
    maxP = max(p);
    
    p_pos = p-minP;
    % p_pos_norm = p_pos / (maxP - minP) * maxP; % Normalize the positive pressures
    
    p_out = p_pos/max(p_pos) * maxP;

    
    
end

== matlab function s20260507_5_PIDAdConfig_IMU_quadleg/MATLAB Function10 ==
  data: dtheta input; p output; dphi input; J input
% function p = config3pressure_projection(dtheta, dphi, J, phi)
% %#codegen
% 
%     p = zeros(3,1);
% 
%     if ~all(isfinite(J), 'all') || ~isfinite(dtheta) || ~isfinite(dphi) || ~isfinite(phi)
%         return;
%     end
% 
%     % Damping schedule
%     lambda_min = 0.01;
%     lambda_max = 0.2;
%     phi_c      = 0.02;
% 
%     lambda = lambda_min + (lambda_max - lambda_min) * exp(-abs(phi)/phi_c);
% 
%     dq = [dtheta; dphi];
%     A = J * J.' + (lambda^2) * eye(2);
% 
%     if rcond(A) < 1e-10
%         return;
%     end
% 
%     p = J.' * (A \ dq);
% 
%     if any(~isfinite(p))
%         p = zeros(3,1);
%     end
% end

function p  = direct_pressure_adaptive(dtheta, dphi, J)
% J: 2x3
% p: 3x1 pressure increment from configuration increment [dtheta; dphi]

p = pinv(J) * [dtheta; dphi]; 

    % lambda = 0.01;   % tune this
    % 
    % dq = [dtheta; dphi];
    % 
    % A = J * J.' + (lambda^2) * eye(2);
    % p = J.' * (A \ dq);
     

end

== matlab function s20260507_5_PIDAdConfig_IMU_quadleg/MATLAB Function4 ==
  data: p input; c output; R output
function [c, R] = pressure2config(p)

A = pi*(0.013/2)^2;
K = 0.27991;
r = 0.0130;

c = [atan2(-A * r * sqrt(0.3e1) * (p(2) - p(3)) / 0.2e1, -A * r * (-p(2) - p(3) + 0.2e1 * p(1)) / 0.2e1), sqrt(A ^ 2 * r ^ 2 * (p(1) ^ 2 - p(2) * p(1) - p(3) * p(1) + p(2) ^ 2 - p(2) * p(3) + p(3) ^ 2)) / K];

R = rank(c);

end

== matlab function s20260507_5_PIDAdConfig_IMU_quadleg/wrap2Pi ==
  data: a input; wa output
function wa = wrap2pi(a)

wa = wrapToPi(a);


end

== matlab function s20260507_5_PIDAdConfig_IMU_quadleg/MATLAB Function7 ==
  data: x input; p output
function p = f20250919_2_InvDeadzone(x)

Pmax = 3e5;
D = [0.5e5; 0.5e5; 0.5e5];
d = [0.1e5; 0.1e5; 0.1e5];

% p = (D .* Pmax - x .* D + x .* Pmax) ./ Pmax ...
%     .* (0.5 .* tanh(1e5 .* x) + 0.5) ...
%     .* (0.5 .* tanh(1e5 .* (Pmax - x)) + 0.5) ...
%     + Pmax .* (-0.5 .* tanh(1e5 .* (Pmax - x)) + 0.5);

p = D ./ d .* x .* (0.5e0 .* tanh((100000 .* x)) + 0.5e0) .* (0.5e0 .* tanh((100000 .* d - 100000 .* x)) + 0.5e0) + ((Pmax - D) ./ (Pmax - d) .* x + (D - d) ./ (Pmax - d) .* Pmax) .* (-0.5e0 .* tanh((100000 .* d - 100000 .* x)) + 0.5e0) .* (0.5e0 .* tanh(0.100000e6 .* Pmax - (100000 .* x)) + 0.5e0) + Pmax .* (-0.5e0 .* tanh(0.100000e6 .* Pmax - (100000 .* x)) + 0.5e0);
if p(1) <= d(1)
    p(1) = D(1);
end
if p(2) <= d(2)
    p(2) = D(2);
end
if p(3) <= d(3)
    p(3) = D(3);
end

end

== matlab function s20260507_5_PIDAdConfig_IMU_quadleg/Adapt parameter ==
  data: dtheta input; p output; dphi input; J input; R output
function [p, R]  = direct_pressure_adaptive(dtheta, dphi, J)
% J: 2x3
% p: 3x1 pressure increment from configuration increment [dtheta; dphi]

p = pinv(J) * [dtheta; dphi]; 

    % lambda = 0.01;   % tune this
    % 
    % dq = [dtheta; dphi];
    % 
    % A = J * J.' + (lambda^2) * eye(2);
    % p = J.' * (A \ dq);

    R = rank(p);
end

% function [p, R] = direct_pressure_adaptive(dtheta, dphi, J, phi)
% %#codegen
% 
%     p = zeros(3,1);
%     R = 0;
% 
%     if ~all(isfinite(J), 'all') || ~isfinite(dtheta) || ~isfinite(dphi) || ~isfinite(phi)
%         return;
%     end
% 
%     % Damping schedule
%     lambda_min = 0.01;
%     lambda_max = 0.2;
%     phi_c      = 0.02;
% 
%     lambda = lambda_min + (lambda_max - lambda_min) * exp(-abs(phi)/phi_c);
% 
%     dq = [dtheta; dphi];
%     A = J * J.' + (lambda^2) * eye(2);
% 
%     if rcond(A) < 1e-10
%         return;
%     end
% 
%     p = J.' * (A \ dq);
% 
%     if any(~isfinite(p))
%         p = zeros(3,1);
%     end
% 
%     R = rank(p);
% end

== matlab function s20260507_5_PIDAdConfig_IMU_quadleg/MATLAB Function3 ==
  data: g input; gad output; phi input
function gad  = PgainAdapt(g, phi)

    min_gain = 0.1;
    max_gain = g;

    gad = min_gain + max_gain / (1 + exp(-(10*phi - 5)));


    
    
end

== matlab function s20260507_5_PIDAdConfig_IMU_quadleg/MATLAB Function6 ==
  data: g input; gad output; phi input
function gad  = PgainAdapt(g, phi)

    min_gain = 0.1;
    max_gain = g;

    gad = min_gain + max_gain / (1 + exp(-(10*phi - 5)));


    
    
end

== matlab function s20260507_5_PIDAdConfig_IMU_quadleg/MATLAB Function2 ==
  data: dtheta input; p output; dphi input; J input
function p  = config3pressure_projection(dtheta, dphi, J)

    p = J \ [dtheta; dphi];
end

== matlab function s20260507_5_PIDAdConfig_IMU_quadleg/PositivePresure ==
  data: p input; p_out output
function p_out  = PositivePressure(p)

    minP = min(p);
    maxP = max(p);
    
    p_pos = p-minP;
    % p_pos_norm = p_pos / (maxP - minP) * maxP; % Normalize the positive pressures
    
    p_out = p_pos/max(p_pos) * maxP;
    
end

== matlab function s20260507_5_PIDAdConfig_IMU_quadleg/Measured theta, phi/MATLAB Function3 ==
  data: s0 input; theta1 output; s1 input; phi1 output; s2 input; s3 input; theta2 output; phi2 output; theta3 output; phi3 output
function [theta1,phi1,theta2,phi2,theta3,phi3]= fcn(s0,s1,s2,s3)

s0_start=[0,0,0,1];
s1_start=[0,0,0,1];
s2_start=[0,0,0,1];
s3_start=[0,0,0,1];


%base=[base1(3),base1(4),base1(5),base1(6)];

sensor0=[s0(6),s0(3),s0(5),s0(4)]; %base
sensor1=[s1(6),s1(3),s1(5),s1(4)];
sensor2=[s2(6),s2(3),s2(5),s2(4)];
sensor3=[s3(6),s3(3),s3(5),s3(4)];

%tip_relative_base=quatmultiply(quatmultiply(tip,quatinv(tip_start)),quatinv(quatmultiply(base,quatinv(base_start))));

sensor1_relative_sensor0=quatmultiply(quatmultiply(sensor1,quatinv(s1_start)),quatinv(quatmultiply(sensor0,quatinv(s0_start))));
sensor2_relative_sensor1=quatmultiply(quatmultiply(sensor2,quatinv(s2_start)),quatinv(quatmultiply(sensor1,quatinv(s1_start))));
sensor3_relative_sensor2=quatmultiply(quatmultiply(sensor3,quatinv(s3_start)),quatinv(quatmultiply(sensor2,quatinv(s2_start))));

%rotMat = quat2tform(tip_relative_base);
rotMat1 = quat2tform(sensor1_relative_sensor0); % only base
theta1= (atan2(rotMat1(2,3),rotMat1(1,3)));
phi1= (acos(rotMat1(3,3)));

rotMat2 = quat2tform(sensor2_relative_sensor1); 
theta2=  (atan2(rotMat2(2,3),rotMat2(1,3)));
phi2= (acos(rotMat2(3,3)));

rotMat3 = quat2tform(sensor3_relative_sensor2); 
theta3= (atan2(rotMat3(2,3),rotMat3(1,3)));
phi3= (acos(rotMat3(3,3)));


end

== matlab function s20260507_5_PIDAdConfig_IMU_quadleg/error cal ==
  data: thetad input; theta_e output; phid input; theta input; phi input; phi_e output
function [theta_e, phi_e]    = fcn(thetad, phid, theta, phi)

    % qd = [thetad;phid];
    % q = [theta;phi];
    % 
    % abs_diff = abs(thetad-theta);
    % abs_diff_mod = abs(mod(thetad, 2*pi)-mod(theta, 2*pi));
    % 
    % if abs_diff < abs_diff_mod
    %     error = qd-q;
    % else
    %     error = mod(qd, 2*pi) - mod(q,2*pi);
    % end
    % 
    % if error(1) < 0.0001
    %     error(1) = 0;
    % end
    % 
    % if error(2) < 0.0001
    %     error(2) = 0;
    % end
    % 
    % theta_e = error(1);
    % phi_e = error(2);

        % Compute signed angular differences in (-pi, pi]
    theta_e = atan2(sin(thetad - theta), cos(thetad - theta));
    phi_e   = atan2(sin(phid - phi), cos(phid - phi));

    % Optional: zero small errors
    if abs(theta_e) < 1e-4
        theta_e = 0;
    end
    if abs(phi_e) < 1e-4
        phi_e = 0;
    end

end

== matlab function s20260507_5_PIDAdConfig_IMU_quadleg/Measured theta, phi/MATLAB Function4 ==
  data: u input; s0 output; a input; b input; c input; d input; e input; s00 input; s11 input; s1 output; s22 input; s33 input; s2 output; s3 output
function [s0,s1,s2,s3]= fcn(u,a,b,c,d,e,s00,s11,s22,s33)
if u==1.0
    %base1=[double(u),double(a),double(b),double(c),double(d),double(e)];
    s00(1)=double(u);
    s00(2)=double(a);
    s00(3)=double(b); %x
    s00(4)=double(c); %y
    s00(5)=double(d); %z
    s00(6)=double(e); %w

elseif u==2.0
    %tip1=[double(u),double(a),double(b),double(c),double(d),double(e)];
    s11(1)=double(u);
    s11(2)=double(a);
    s11(3)=double(b);
    s11(4)=double(c);
    s11(5)=double(d);
    s11(6)=double(e);
elseif u==3.0
    %tip1=[double(u),double(a),double(b),double(c),double(d),double(e)];
    s22(1)=double(u);
    s22(2)=double(a);
    s22(3)=double(b);
    s22(4)=double(c);
    s22(5)=double(d);
    s22(6)=double(e);
elseif u==4.0
    %tip1=[double(u),double(a),double(b),double(c),double(d),double(e)];
    s33(1)=double(u);
    s33(2)=double(a);
    s33(3)=double(b);
    s33(4)=double(c);
    s33(5)=double(d);
    s33(6)=double(e);
end
    s0=s00;
    s1=s11;
    s2=s22;
    s3=s33;

end
